simulink model "q1"  (R2017a)
settings: Solver=FixedStepDiscrete  StartTime=0.0  StopTime=5.0  RelTol=1e-3
values from neighbouring files (symbols this model uses):
  C = [1 0]    [workspace.m]
  F = [f1 f2]    [workspace.m]
  G = [[0.5 1]; [0.5 0.7]]    [workspace.m]
  H1 = [0.2; 0.1]    [workspace.m]
  H2 = [1; 0]    [workspace.m]
  N = 1/(C * inv(eye(2) - G + H1*F) * H1)    [workspace.m]
settings Model: Creator=arthur  LastModifiedBy=arthur

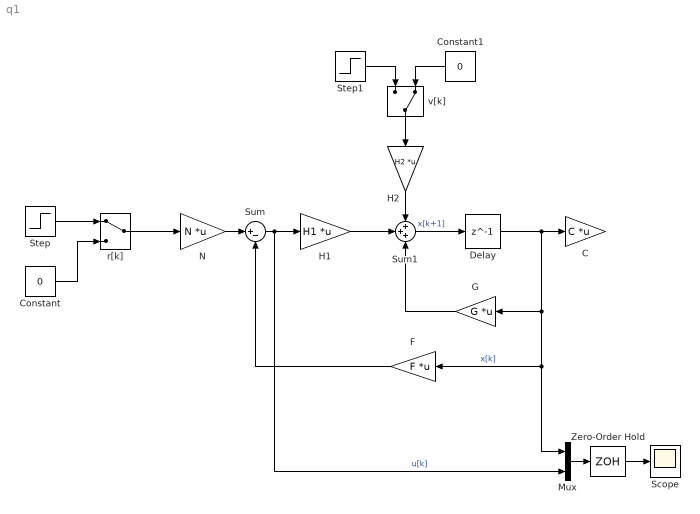
== system q1 ==
  C : Gain  Gain=C  Multiplication=Matrix(K*u)
  Constant : Constant  Value=0
  Constant1 : Constant  Value=0
  Delay : Delay  DelayLength=1  InitialCondition=0
  F : Gain  Gain=F  Multiplication=Matrix(K*u)
  G : Gain  Gain=G  Multiplication=Matrix(K*u)
  H1 : Gain  Gain=H1  Multiplication=Matrix(K*u)
  H2 : Gain  Gain=H2  Multiplication=Matrix(K*u)
  Mux : Mux  Inputs=2
  N : Gain  Gain=N  Multiplication=Matrix(K*u)
  Scope : Scope
  Step : Step  Time=0  SampleTime=0
  Step1 : Step  Time=0  SampleTime=0
  Sum : Sum  Inputs=|+-
  Sum1 : Sum  Inputs=+++
  Zero-Order Hold : ZeroOrderHold  SampleTime=-1
  r[k] : ManualSwitch
  v[k] : ManualSwitch  CurrentSetting=0
  wires:
  r[k]/1 -> N/1
  N/1 -> Sum/1
  Sum/1 -> Mux/2, H1/1  "u[k]"
  H2/1 -> Sum1/1
  H1/1 -> Sum1/2
  v[k]/1 -> H2/1
  Sum1/1 -> Delay/1  "x[k+1]"
  Delay/1 -> C/1, G/1, Mux/1, F/1  "x[k]"
  G/1 -> Sum1/3
  F/1 -> Sum/2
  Step1/1 -> v[k]/1
  Step/1 -> r[k]/1
  Constant/1 -> r[k]/2
  Constant1/1 -> v[k]/2
  Mux/1 -> Zero-Order Hold/1
  Zero-Order Hold/1 -> Scope/1
